simulink model "DTMF_Telefonie_Project_Crehul_Hornai"  (R2018b)
settings: Solver=VariableStepAuto  StartTime=0.0  StopTime=100  RelTol=1e-3
undefined symbols (not defined in the file): fdesignblkfcn, gcbh
libraries: simulink x12, dspfdesign x7
(part 1 of 4)
settings Model: Creator=vladc  LastModifiedBy=vladc

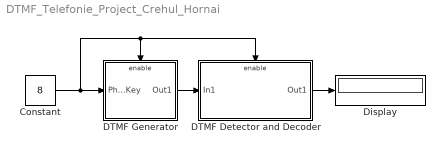
== system DTMF_Telefonie_Project_Crehul_Hornai ==
  Constant : Constant  Value=8  SampleTime=0.00001
  DTMF Detector and Decoder : Subsystem
  DTMF Generator : Subsystem
  Display : Display
      settings: Format=decimal (Stored Integer)
  wires:
  Constant/1 -> DTMF Detector and Decoder/Enable, DTMF Generator/Enable, DTMF Generator/1(PhoneKey)
  DTMF Generator/1(Out1) -> DTMF Detector and Decoder/1(In1)
  DTMF Detector and Decoder/1(Out1) -> Display/1

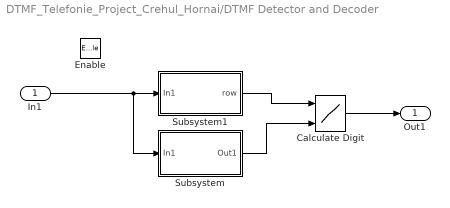
== system DTMF_Telefonie_Project_Crehul_Hornai/DTMF Detector and Decoder ==
  In1 : Inport
  Enable : EnablePort
  Calculate Digit : Lookup_n-D  BreakpointsForDimension1=[1:4]  BreakpointsForDimension2=[1:3]  Table=[1 2 3;4 5 6;7 8 9;10 0 11]  ExtrapMethod=Clip  SaturateOnIntegerOverflow=on  InputSameDT=on
  Subsystem : Subsystem
  Subsystem1 : Subsystem
  Out1 : Outport
  wires:
  In1/1 -> Subsystem/1(In1), Subsystem1/1(In1)
  Calculate Digit/1 -> Out1/1
  Subsystem1/1(row) -> Calculate Digit/1
  Subsystem/1(Out1) -> Calculate Digit/2

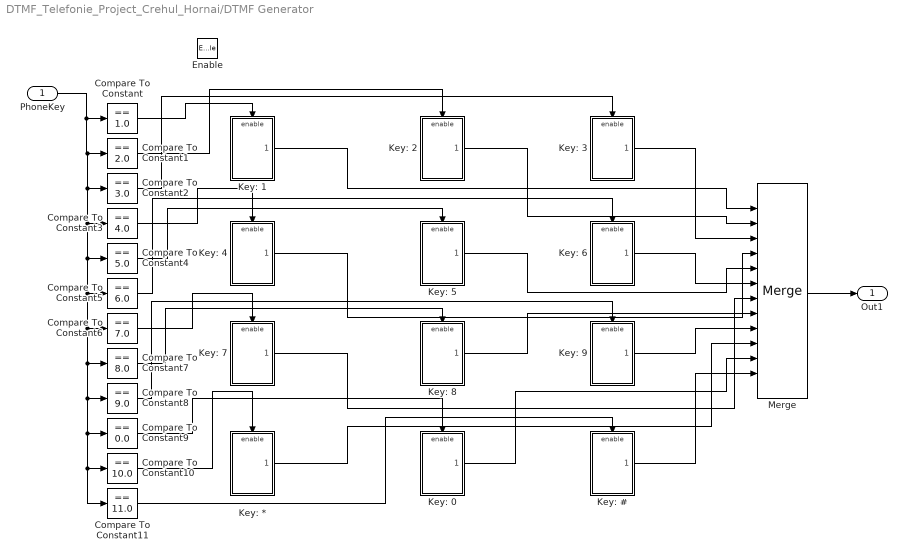
== system DTMF_Telefonie_Project_Crehul_Hornai/DTMF Generator ==
  PhoneKey : Inport
  Enable : EnablePort
  Compare To Constant : simulink/Logic and Bit Operations/Compare To Constant  relop===  const=1.0  OutDataTypeStr=boolean
  Compare To Constant1 : simulink/Logic and Bit Operations/Compare To Constant  relop===  const=2.0  OutDataTypeStr=boolean
  Compare To Constant10 : simulink/Logic and Bit Operations/Compare To Constant  relop===  const=10.0  OutDataTypeStr=boolean
  Compare To Constant11 : simulink/Logic and Bit Operations/Compare To Constant  relop===  const=11.0  OutDataTypeStr=boolean
  Compare To Constant2 : simulink/Logic and Bit Operations/Compare To Constant  relop===  const=3.0  OutDataTypeStr=boolean
  Compare To Constant3 : simulink/Logic and Bit Operations/Compare To Constant  relop===  const=4.0  OutDataTypeStr=boolean
  Compare To Constant4 : simulink/Logic and Bit Operations/Compare To Constant  relop===  const=5.0  OutDataTypeStr=boolean
  Compare To Constant5 : simulink/Logic and Bit Operations/Compare To Constant  relop===  const=6.0  OutDataTypeStr=boolean
  Compare To Constant6 : simulink/Logic and Bit Operations/Compare To Constant  relop===  const=7.0  OutDataTypeStr=boolean
  Compare To Constant7 : simulink/Logic and Bit Operations/Compare To Constant  relop===  const=8.0  OutDataTypeStr=boolean
  Compare To Constant8 : simulink/Logic and Bit Operations/Compare To Constant  relop===  const=9.0  OutDataTypeStr=boolean
  Compare To Constant9 : simulink/Logic and Bit Operations/Compare To Constant  relop===  const=0.0  OutDataTypeStr=boolean
  Key: # : Subsystem
  Key: * : Subsystem
  Key: 0 : Subsystem
  Key: 1 : Subsystem
  Key: 2 : Subsystem
  Key: 3 : Subsystem
  Key: 4 : Subsystem
  Key: 5 : Subsystem
  Key: 6 : Subsystem
  Key: 7 : Subsystem
  Key: 8 : Subsystem
  Key: 9 : Subsystem
  Merge : Merge  Inputs=12
  Out1 : Outport
  wires:
  Key: 7/1(Out_Button_3) -> Merge/7
  PhoneKey/1 -> Compare To Constant11/1, Compare To Constant10/1, Compare To Constant9/1, Compare To Constant8/1, Compare To Constant7/1, Compare To Constant6/1, Compare To Constant5/1, Compare To Constant4/1, Compare To Constant3/1, Compare To Constant2/1, Compare To Constant1/1, Compare To Constant/1
  Compare To Constant6/1 -> Key: 7/Enable
  Key: 1/1(Out_Button_1) -> Merge/1
  Merge/1 -> Out1/1
  Compare To Constant3/1 -> Key: 4/Enable
  Key: 3/1(Out_Button_8) -> Merge/3
  Key: 8/1(Out_Button_7) -> Merge/8
  Compare To Constant4/1 -> Key: 5/Enable
  Key: 0/1(Out_Button_9) -> Merge/11
  Compare To Constant11/1 -> Key: #/Enable
  Compare To Constant/1 -> Key: 1/Enable
  Compare To Constant2/1 -> Key: 3/Enable
  Key: 9/1(Out_Button_11) -> Merge/9
  Compare To Constant9/1 -> Key: 0/Enable
  Compare To Constant10/1 -> Key: */Enable
  Key: 5/1(Out_Button_6) -> Merge/5
  Key: 2/1(Out_Button_5) -> Merge/2
  Key: 6/1(Out_Button_10) -> Merge/6
  Compare To Constant7/1 -> Key: 8/Enable
  Key: */1(Out_Button_4) -> Merge/10
  Compare To Constant5/1 -> Key: 6/Enable
  Compare To Constant8/1 -> Key: 9/Enable
  Compare To Constant1/1 -> Key: 2/Enable
  Key: #/1(Out_Button_12) -> Merge/12
  Key: 4/1(Out_Button_2) -> Merge/4

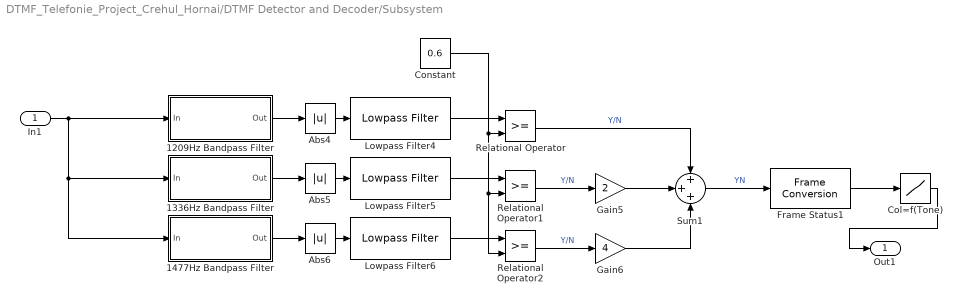
== system DTMF_Telefonie_Project_Crehul_Hornai/DTMF Detector and Decoder/Subsystem ==
  In1 : Inport
  1209Hz Bandpass Filter : Subsystem  DialogController=fdesignblkfcn  InitFcn=fdesignblkfcn(gcbh, {'InitFcn'});  mask(Bandpass Filter){}
      mask help: Design a bandpass filter
      settings: CopyFcn=fdesignblkfcn(gcbh, {'CopyFcn'});
      mask Help: helpview(mapfilelocation('dsp'), 'dspbandpassfilter');
      mask Display: disp('Bandpass');
  1336Hz Bandpass Filter : Subsystem  DialogController=fdesignblkfcn  InitFcn=fdesignblkfcn(gcbh, {'InitFcn'});  mask(Bandpass Filter){}
      mask help: Design a bandpass filter
      settings: CopyFcn=fdesignblkfcn(gcbh, {'CopyFcn'});
      mask Help: helpview(mapfilelocation('dsp'), 'dspbandpassfilter');
      mask Display: disp('Bandpass');
  1477Hz Bandpass Filter : Subsystem  DialogController=fdesignblkfcn  InitFcn=fdesignblkfcn(gcbh, {'InitFcn'});  mask(Bandpass Filter){}
      mask help: Design a bandpass filter
      settings: CopyFcn=fdesignblkfcn(gcbh, {'CopyFcn'});
      mask Help: helpview(mapfilelocation('dsp'), 'dspbandpassfilter');
      mask Display: disp('Bandpass');
  Abs4 : Abs
  Abs5 : Abs
  Abs6 : Abs
  Col=f(Tone) : Lookup_n-D  NumberOfTableDimensions=1  BreakpointsForDimension1=[0:7]  Table=[0 1 2 0 3 0 0 0]  ExtrapMethod=Clip  SaturateOnIntegerOverflow=on  InputSameDT=on
  Constant : Constant  Value=0.6
  Frame Status1 : FrameConversion  OutFrame=Sample-based
  Gain5 : Gain  Gain=2
  Gain6 : Gain  Gain=4
  Lowpass Filter4 : dspfdesign/Lowpass Filter  FilterType=FIR  DesignForMinimumOrder=on  FilterOrder=50  PassbandFrequency=100  StopbandFrequency=130  PassbandRipple=0.1  StopbandAttenuation=80  InheritSampleRate=on  SampleRate=44100  SimulateUsing=Interpreted execution  roundingMode=Floor  coeffsDataTypeStr=fixdt(1,16)
  Lowpass Filter5 : dspfdesign/Lowpass Filter  FilterType=FIR  DesignForMinimumOrder=on  FilterOrder=50  PassbandFrequency=100  StopbandFrequency=130  PassbandRipple=0.1  StopbandAttenuation=80  InheritSampleRate=on  SampleRate=44100  SimulateUsing=Interpreted execution  roundingMode=Floor  coeffsDataTypeStr=fixdt(1,16)
  Lowpass Filter6 : dspfdesign/Lowpass Filter  FilterType=FIR  DesignForMinimumOrder=on  FilterOrder=50  PassbandFrequency=100  StopbandFrequency=130  PassbandRipple=0.1  StopbandAttenuation=80  InheritSampleRate=on  SampleRate=44100  SimulateUsing=Interpreted execution  roundingMode=Floor  coeffsDataTypeStr=fixdt(1,16)
  Relational Operator : RelationalOperator  RndMeth=Nearest  InputSameDT=on
  Relational Operator1 : RelationalOperator  RndMeth=Nearest  InputSameDT=on
  Relational Operator2 : RelationalOperator  RndMeth=Nearest  InputSameDT=on
  Sum1 : Sum  Inputs=+++
  Out1 : Outport
  wires:
  Abs4/1 -> Lowpass Filter4/1
  1336Hz Bandpass Filter/1(Out) -> Abs5/1
  In1/1 -> 1477Hz Bandpass Filter/1(In), 1336Hz Bandpass Filter/1(In), 1209Hz Bandpass Filter/1(In)
  Abs6/1 -> Lowpass Filter6/1
  Abs5/1 -> Lowpass Filter5/1
  1209Hz Bandpass Filter/1(Out) -> Abs4/1
  1477Hz Bandpass Filter/1(Out) -> Abs6/1
  Gain5/1 -> Sum1/2
  Gain6/1 -> Sum1/3
  Sum1/1 -> Frame Status1/1  "YN"
  Frame Status1/1 -> Col=f(Tone)/1
  Col=f(Tone)/1 -> Out1/1
  Lowpass Filter4/1 -> Relational Operator/1
  Lowpass Filter5/1 -> Relational Operator1/1
  Lowpass Filter6/1 -> Relational Operator2/1
  Constant/1 -> Relational Operator2/2, Relational Operator1/2, Relational Operator/2
  Relational Operator/1 -> Sum1/1  "Y/N"
  Relational Operator1/1 -> Gain5/1  "Y/N"
  Relational Operator2/1 -> Gain6/1  "Y/N"

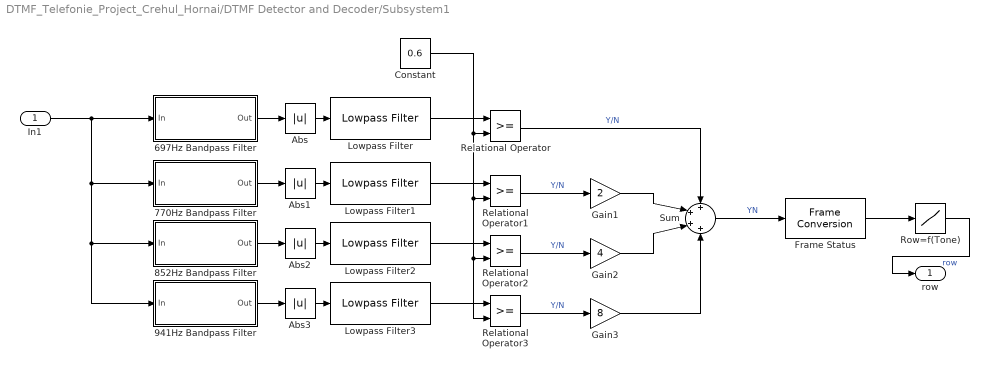
== system DTMF_Telefonie_Project_Crehul_Hornai/DTMF Detector and Decoder/Subsystem1 ==
  In1 : Inport
  697Hz Bandpass Filter : Subsystem  DialogController=fdesignblkfcn  InitFcn=fdesignblkfcn(gcbh, {'InitFcn'});  mask(Bandpass Filter){}
      mask help: Design a bandpass filter
      settings: CopyFcn=fdesignblkfcn(gcbh, {'CopyFcn'});
      mask Help: helpview(mapfilelocation('dsp'), 'dspbandpassfilter');
      mask Display: disp('Bandpass');
  770Hz Bandpass Filter : Subsystem  DialogController=fdesignblkfcn  InitFcn=fdesignblkfcn(gcbh, {'InitFcn'});  mask(Bandpass Filter){}
      mask help: Design a bandpass filter
      settings: CopyFcn=fdesignblkfcn(gcbh, {'CopyFcn'});
      mask Help: helpview(mapfilelocation('dsp'), 'dspbandpassfilter');
      mask Display: disp('Bandpass');
  852Hz Bandpass Filter : Subsystem  DialogController=fdesignblkfcn  InitFcn=fdesignblkfcn(gcbh, {'InitFcn'});  mask(Bandpass Filter){}
      mask help: Design a bandpass filter
      settings: CopyFcn=fdesignblkfcn(gcbh, {'CopyFcn'});
      mask Help: helpview(mapfilelocation('dsp'), 'dspbandpassfilter');
      mask Display: disp('Bandpass');
  941Hz Bandpass Filter : Subsystem  DialogController=fdesignblkfcn  InitFcn=fdesignblkfcn(gcbh, {'InitFcn'});  mask(Bandpass Filter){}
      mask help: Design a bandpass filter
      settings: CopyFcn=fdesignblkfcn(gcbh, {'CopyFcn'});
      mask Help: helpview(mapfilelocation('dsp'), 'dspbandpassfilter');
      mask Display: disp('Bandpass');
  Abs{,1..3} (4 alike) : Abs
  Constant : Constant  Value=0.6
  Frame Status : FrameConversion  OutFrame=Sample-based
  Gain1 : Gain  Gain=2
  Gain2 : Gain  Gain=4
  Gain3 : Gain  Gain=8
  Lowpass Filter : dspfdesign/Lowpass Filter  FilterType=IIR  DesignForMinimumOrder=on  FilterOrder=50  PassbandFrequency=100  StopbandFrequency=230  PassbandRipple=0.1  StopbandAttenuation=20  InheritSampleRate=off  SampleRate=44100  SimulateUsing=Interpreted execution  roundingMode=Floor  coeffsDataTypeStr=fixdt(1,16)
  Lowpass Filter1 : dspfdesign/Lowpass Filter  FilterType=FIR  DesignForMinimumOrder=on  FilterOrder=50  PassbandFrequency=100  StopbandFrequency=130  PassbandRipple=0.1  StopbandAttenuation=80  InheritSampleRate=on  SampleRate=44100  SimulateUsing=Interpreted execution  roundingMode=Floor  coeffsDataTypeStr=fixdt(1,16)
  Lowpass Filter2 : dspfdesign/Lowpass Filter  FilterType=FIR  DesignForMinimumOrder=on  FilterOrder=50  PassbandFrequency=100  StopbandFrequency=130  PassbandRipple=0.1  StopbandAttenuation=80  InheritSampleRate=on  SampleRate=44100  SimulateUsing=Interpreted execution  roundingMode=Floor  coeffsDataTypeStr=fixdt(1,16)
  Lowpass Filter3 : dspfdesign/Lowpass Filter  FilterType=FIR  DesignForMinimumOrder=on  FilterOrder=50  PassbandFrequency=100  StopbandFrequency=130  PassbandRipple=0.1  StopbandAttenuation=80  InheritSampleRate=on  SampleRate=44100  SimulateUsing=Interpreted execution  roundingMode=Floor  coeffsDataTypeStr=fixdt(1,16)
  Relational Operator{,1..3} (4 alike) : RelationalOperator  RndMeth=Nearest  InputSameDT=on
  Row=f(Tone) : Lookup_n-D  NumberOfTableDimensions=1  BreakpointsForDimension1=[0:15]  Table=[0 1 2 0 3 0 0 0 4 0 0 0 0 0 0 0]  ExtrapMethod=Clip  SaturateOnIntegerOverflow=on  InputSameDT=on
  Sum : Sum  Inputs=++++
  row : Outport
  wires:
  Sum/1 -> Frame Status/1  "YN"
  Abs/1 -> Lowpass Filter/1
  Abs1/1 -> Lowpass Filter1/1
  770Hz Bandpass Filter/1(Out) -> Abs1/1
  697Hz Bandpass Filter/1(Out) -> Abs/1
  Abs3/1 -> Lowpass Filter3/1
  Gain2/1 -> Sum/3
  Frame Status/1 -> Row=f(Tone)/1
  Gain3/1 -> Sum/4
  Abs2/1 -> Lowpass Filter2/1
  852Hz Bandpass Filter/1(Out) -> Abs2/1
  941Hz Bandpass Filter/1(Out) -> Abs3/1
  Gain1/1 -> Sum/2
  In1/1 -> 941Hz Bandpass Filter/1(In), 852Hz Bandpass Filter/1(In), 770Hz Bandpass Filter/1(In), 697Hz Bandpass Filter/1(In)
  Row=f(Tone)/1 -> row/1  "row"
  Lowpass Filter/1 -> Relational Operator/1
  Lowpass Filter1/1 -> Relational Operator1/1
  Lowpass Filter2/1 -> Relational Operator2/1
  Lowpass Filter3/1 -> Relational Operator3/1
  Constant/1 -> Relational Operator3/2, Relational Operator2/2, Relational Operator1/2, Relational Operator/2
  Relational Operator/1 -> Sum/1  "Y/N"
  Relational Operator1/1 -> Gain1/1  "Y/N"
  Relational Operator2/1 -> Gain2/1  "Y/N"
  Relational Operator3/1 -> Gain3/1  "Y/N"

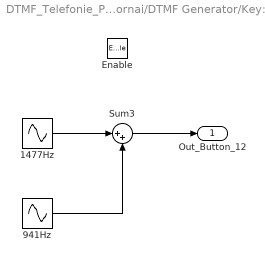
== system DTMF_Telefonie_Project_Crehul_Hornai/DTMF Generator/Key: # ==
  Enable : EnablePort
  1477Hz : Sin  Frequency=1477 * 2 * pi  SampleTime=0.0001
  941Hz : Sin  Frequency=941 * 2 * pi  SampleTime=0.0001
  Sum3 : Sum  Inputs=|++
  Out_Button_12 : Outport
  wires:
  1477Hz/1 -> Sum3/1
  Sum3/1 -> Out_Button_12/1
  941Hz/1 -> Sum3/2

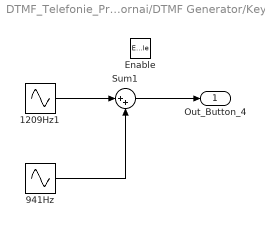
== system DTMF_Telefonie_Project_Crehul_Hornai/DTMF Generator/Key: * ==
  Enable : EnablePort
  1209Hz1 : Sin  Frequency=1209 * 2 * pi  SampleTime=0.0001
  941Hz : Sin  Frequency=941 * 2 * pi  SampleTime=0.0001
  Sum1 : Sum  Inputs=|++
  Out_Button_4 : Outport
  wires:
  941Hz/1 -> Sum1/2
  Sum1/1 -> Out_Button_4/1
  1209Hz1/1 -> Sum1/1

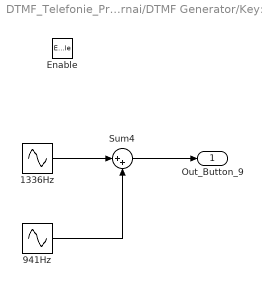
== system DTMF_Telefonie_Project_Crehul_Hornai/DTMF Generator/Key: 0 ==
  Enable : EnablePort
  1336Hz : Sin  Frequency=1336 * 2 * pi  SampleTime=0.0001
  941Hz : Sin  Frequency=941 * 2 * pi  SampleTime=0.0001
  Sum4 : Sum  Inputs=|++
  Out_Button_9 : Outport
  wires:
  1336Hz/1 -> Sum4/1
  Sum4/1 -> Out_Button_9/1
  941Hz/1 -> Sum4/2

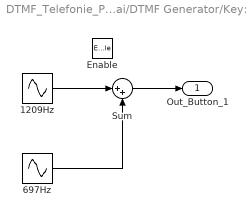
== system DTMF_Telefonie_Project_Crehul_Hornai/DTMF Generator/Key: 1 ==
  Enable : EnablePort
  1209Hz : Sin  Frequency=1209*2*pi  SampleTime=0.0001
  697Hz : Sin  Frequency=697*2*pi  SampleTime=0.0001
  Sum : Sum  Inputs=|++
  Out_Button_1 : Outport
  wires:
  Sum/1 -> Out_Button_1/1
  1209Hz/1 -> Sum/1
  697Hz/1 -> Sum/2

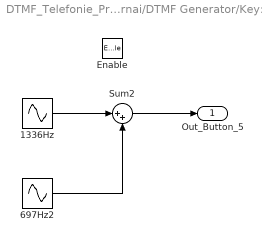
== system DTMF_Telefonie_Project_Crehul_Hornai/DTMF Generator/Key: 2 ==
  Enable : EnablePort
  1336Hz : Sin  Frequency=1336 * 2 * pi  SampleTime=0.0001
  697Hz2 : Sin  Frequency=697 * 2 * pi  SampleTime=0.0001
  Sum2 : Sum  Inputs=|++
  Out_Button_5 : Outport
  wires:
  1336Hz/1 -> Sum2/1
  697Hz2/1 -> Sum2/2
  Sum2/1 -> Out_Button_5/1

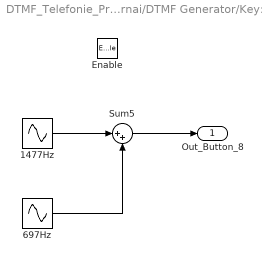
== system DTMF_Telefonie_Project_Crehul_Hornai/DTMF Generator/Key: 3 ==
  Enable : EnablePort
  1477Hz : Sin  Frequency=1477 * 2 * pi  SampleTime=0.0001
  697Hz : Sin  Frequency=697 * 2 * pi  SampleTime=0.0001
  Sum5 : Sum  Inputs=|++
  Out_Button_8 : Outport
  wires:
  697Hz/1 -> Sum5/2
  1477Hz/1 -> Sum5/1
  Sum5/1 -> Out_Button_8/1

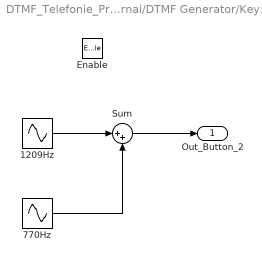
== system DTMF_Telefonie_Project_Crehul_Hornai/DTMF Generator/Key: 4 ==
  Enable : EnablePort
  1209Hz : Sin  Frequency=1209 * 2 * pi  SampleTime=0.0001
  770Hz : Sin  Frequency=770 * 2 * pi  SampleTime=0.0001
  Sum : Sum  Inputs=|++
  Out_Button_2 : Outport
  wires:
  770Hz/1 -> Sum/2
  Sum/1 -> Out_Button_2/1
  1209Hz/1 -> Sum/1

== system DTMF_Telefonie_Project_Crehul_Hornai/DTMF Generator/Key: 5 ==
  Enable : EnablePort
  1336Hz : Sin  Frequency=1336 * 2 * pi  SampleTime=0.0001
  770Hz : Sin  Frequency=770 * 2 * pi  SampleTime=0.0001
  Sum1 : Sum  Inputs=|++
  Out_Button_6 : Outport
  wires:
  Sum1/1 -> Out_Button_6/1
  1336Hz/1 -> Sum1/1
  770Hz/1 -> Sum1/2

== system DTMF_Telefonie_Project_Crehul_Hornai/DTMF Generator/Key: 6 ==
  Enable : EnablePort
  1477Hz : Sin  Frequency=1477 * 2 * pi  SampleTime=0.0001
  770Hz : Sin  Frequency=770 * 2 * pi  SampleTime=0.0001
  Sum1 : Sum  Inputs=|++
  Out_Button_10 : Outport
  wires:
  Sum1/1 -> Out_Button_10/1
  770Hz/1 -> Sum1/2
  1477Hz/1 -> Sum1/1

== system DTMF_Telefonie_Project_Crehul_Hornai/DTMF Generator/Key: 7 ==
  Enable : EnablePort
  1209Hz : Sin  Frequency=1209 * 2 * pi  SampleTime=0.0001
  852Hz : Sin  Frequency=852 * 2 * pi  SampleTime=0.0001
  Sum : Sum  Inputs=|++
  Out_Button_3 : Outport
  wires:
  Sum/1 -> Out_Button_3/1
  852Hz/1 -> Sum/2
  1209Hz/1 -> Sum/1

== system DTMF_Telefonie_Project_Crehul_Hornai/DTMF Generator/Key: 8 ==
  Enable : EnablePort
  1336Hz : Sin  Frequency=1336 * 2 * pi  SampleTime=0.0001
  852Hz : Sin  Frequency=852 * 2 * pi  SampleTime=0.0001
  Sum3 : Sum  Inputs=|++
  Out_Button_7 : Outport
  wires:
  Sum3/1 -> Out_Button_7/1
  852Hz/1 -> Sum3/2
  1336Hz/1 -> Sum3/1

== system DTMF_Telefonie_Project_Crehul_Hornai/DTMF Generator/Key: 9 ==
  Enable : EnablePort
  1477Hz : Sin  Frequency=1477 * 2 * pi  SampleTime=0.0001
  852Hz : Sin  Frequency=852 * 2 * pi  SampleTime=0.0001
  Sum2 : Sum  Inputs=|++
  Out_Button_11 : Outport
  wires:
  1477Hz/1 -> Sum2/1
  Sum2/1 -> Out_Button_11/1
  852Hz/1 -> Sum2/2

== system DTMF_Telefonie_Project_Crehul_Hornai/DTMF Detector and Decoder/Subsystem/1209Hz Bandpass Filter ==
  In : Inport
  Generated Filter Block : DiscreteFir  Tag=BlockMethodSubSystem  Coefficients=[-2.68104316978609227e-05 0.00129524575984109411 0.00027035870583339049 5.97789327057972764e-05 -0.000186064770865025783 -0.00035242675260704643 -0.00033730719511808685 -0.000133492167968419584 0.000159313649341999127 0.00038325330956582161 0.000409612137923090003 0.000213665303268456824 -0.000105208368705157198 -0.000375504388487337922 -0.000447981600112808153 -0.00028128556838711476 3.38150174142128404e-05 0.000324460254122310807 0.000434505373581626424 0.00031190779922032777 3.57001760766895247e-05 -0.000234894518635577658 -0.000355074035898198621 -0.000278061732510660005 -7.37232060620382403e-05 0.00012351148872090335 0.000204887203834534922 0.000153229628683929087 4.43627702712274911e-05 -1.93364116085655968e-05 9.61352545337233223e-06 8.2200891844584666e-05 9.11139960740093863e-05 -3.86869953840555773e-05 -0.000267270539791579281 -0.00043845600455714106 -0.000371517110085582279 -2.57525838629857166e-06 0.000527178747208640773 0.000906762135499263478 0.00082799526502203534 0.000197555808858237633 -0.000736341130457315472 -0.0014631876531442775 -0.00147445872959586473 -0.00060054746165218143 0.000825681716434705166 0.0020556208752338526 0.00231091693758213182 0.00125685357644432115 -0.000720825763344560546 -0.00261642376123233898 -0.00330660983458850406 -0.00219625239510655868 0.000345082450964913118 0.0030589828511720994 0.00440537932230107912 0.00342364119313599662 0.000367194158988320496 -0.00328404793730521912 -0.00552483957470165619 -0.00491298865833330288 -0.00146411400584531997 0.00319144848899657278 0.00655873909436608532 0.00660593914431226777 0.00296540050227270388 -0.00268831680978220749 -0.00738475389415002396 -0.00840901501835418334 -0.00485507173627933251 0.00170278816863107113 0.00787443560336700474 0.0102000406479683427 0.00707754650524016968 -0.000192530533589101833 -0.00790609243381684527 -0.011834345331829723 -0.00953686701253677813 -0.00184357313558901727 0.00737717047285702497 0.0131563591006881898 0.0120995191776441663 0.00436243607936683681 -0.00621715218472063385 -0.0140129083683532656 -0.0146038901566436091 -0.00727232734794326999 0.0043988233791988976 0.0142683352181379036 0.0168697925287066217 0.0104383454868257012 -0.00194538476620552186 -0.013819268353057506 -0.0187150214165393292 -0.013688095887563867 -0.00106668380659103671 0.0126060087320333143 0.0199712647995053949 0.016824321031839895 0.00450931037998957961 -0.0106235729079248737 -0.0204996344955463462 -0.0196414793671116292 -0.00821005216197508332 0.00792476375210000687 0.0202056230547902754 0.0219417901625978823 0.0119644253196142109 -0.00462002904940317372 -0.0190496505763591353 -0.0235536478981206096 -0.0155516191114862881 0.000870680881692380108 0.0170536701314248883 0.0243468151315176726 0.0187524534348275582 0.00312196837493620158 -0.0143009154233129654 -0.0242455404107973886 -0.0213677785659719052 -0.00713308143887335291 0.0109319443381326528 0.0232357829412106198 0.0232357829412106198 0.0109319443381326528 -0.00713308143887335291 -0.0213677785659719052 -0.0242455404107973886 -0.0143009154233129654 0.00312196837493620158 0.0187524534348275582 0.0243468151315176726 0.0170536701314248883 0.000870680881692380108 -0.0155516191114862881 -0.0235536478981206096 -0.0190496505763591353 -0.00462002904940317372 0.0119644253196142109 0.0219417901625978823 0.0202056230547902754 0.00792476375210000687 -0.00821005216197508332 -0.0196414793671116292 -0.0204996344955463462 -0.0106235729079248737 0.00450931037998957961 0.016824321031839895 0.0199712647995053949 0.0126060087320333143 -0.00106668380659103671 -0.013688095887563867 -0.0187150214165393292 -0.013819268353057506 -0.00194538476620552186 0.0104383454868257012 0.0168697925287066217 0.0142683352181379036 0.0043988233791988976 -0.00727232734794326999 -0.0146038901566436091 -0.0140129083683532656 -0.00621715218472063385 0.00436243607936683681 0.0120995191776441663 0.0131563591006881898 0.00737717047285702497 -0.00184357313558901727 -0.00953686701253677813 -0.011834345331829723 ...(+1841 chars)]  InputProcessing=Columns as channels (frame based)
  Out : Outport
  wires:
  In/1 -> Generated Filter Block/1
  Generated Filter Block/1 -> Out/1

== system DTMF_Telefonie_Project_Crehul_Hornai/DTMF Detector and Decoder/Subsystem/1336Hz Bandpass Filter ==
  In : Inport
  Generated Filter Block : DiscreteFir  Tag=BlockMethodSubSystem  Coefficients=[2.69394371099855751e-06 0.00117165562921208344 6.3491850840960342e-05 -8.4624399806407756e-06 -7.99037446358266158e-05 -0.000100868926562373102 -5.44997145059411287e-05 2.99848082026595714e-05 9.79779952662868797e-05 0.000102408748187840688 3.8591008586048468e-05 -5.38855233033176065e-05 -0.000113249385257364584 -9.91491147698982112e-05 -1.76735024774710408e-05 7.81776597637631743e-05 0.000125321473120212782 8.97261386021443435e-05 -6.84389521436474385e-06 -0.000102423933573247061 -0.000132194500866850573 -7.47793614721613091e-05 3.48838671897974944e-05 0.000124265245919175787 0.000133612318573405036 5.35064240703645843e-05 -6.43653826217515952e-05 -0.000142970502120994382 -0.000127873321259458191 -2.73088738157248323e-05 9.45644837702661403e-05 0.000156116735515599145 0.000115425698771689112 -3.70090411639474245e-06 -0.000122933802227524844 -0.000163503928826842218 -9.56295760272910401e-05 3.72712863555299621e-05 0.000149025673371245377 0.000163778588022141236 7.01447106457836044e-05 -7.31253099060873938e-05 -0.000170820259461797229 -0.000157595910391976606 -3.84203641555552668e-05 0.000108265265782551317 0.000186014216685199485 0.000139784366467252596 2.54228694596711317e-06 -0.000141708018935495037 -0.000193703904114099707 -0.000117634172643367625 3.76855386470891472e-05 0.000170912899901319538 0.00019282381288382314 8.69878828140518544e-05 -7.8389945689166839e-05 -0.000194479288599821781 -0.000183199077448570552 -5.02045703261934807e-05 0.000118259217613198844 0.000210623481853642984 0.000164701338875474293 8.73055212596081549e-06 -0.000155018157185409693 -0.000218284554096782359 -0.000137486464077824595 3.52799719571198628e-05 0.000186866881074920213 0.000216201526264954424 0.000102804504377550319 -8.00098318612673959e-05 -0.000211482407583856455 -0.000204360174023499605 -6.17691413268889235e-05 0.000122725198727849242 0.000227685078966525199 0.000182713152657773071 1.67753236851202799e-05 -0.000161565278681012961 -0.000234150769841028191 -0.000152639407700760508 3.0332502399682288e-05 0.000194097650494409919 0.000230632166633668164 0.000114920890391796661 -7.68823833482269823e-05 -0.000218563441804632335 -0.000216183825558373399 -7.13433791556549769e-05 0.000120751682992005938 0.000233377503057401615 0.000192508399706572617 2.48156964049557009e-05 -0.000159397689931879563 -0.000237979533786486291 -0.000159788876706973846 2.29484351225081856e-05 0.000190522502272507917 0.00023167990789653794 0.000120748478138963918 -6.92943979297238038e-05 -0.000212397762841430885 -0.000215371893154697562 -7.66656581665382635e-05 0.000110994915730187101 0.000224468546324539881 0.000189426814851585213 3.08040640945889555e-05 -0.000146479066566603932 -0.000225473033556930578 -0.000156045409631158909 1.47784474854167902e-05 0.000173213119583249088 0.000216116279365059435 0.000116843378449837162 -5.67977950993890299e-05 -0.000190310363448117914 -0.000196786541266158205 -7.49770548206403747e-05 9.32354527198771005e-05 0.000196623409868828918 0.000169673649135869365 3.2817692787847361e-05 -0.000121481738994366675 -0.000192623660969485364 -0.000136337989629350953 6.44294111745713494e-06 0.000140439368990387522 0.000178501959768861355 9.97765686525447452e-05 -4.05829609781086648e-05 -0.000148761926126928477 -0.000156468179317936253 -6.27785878042827743e-05 6.66565411803262536e-05 0.000146855225949184048 0.000128144911822030381 2.8422048619754876e-05 -8.36632672263093197e-05 -0.000134813266803125503 -9.67845224833618466e-05 4.76836132450508474e-07 8.99481120179559598e-05 0.000114987091168748971 6.50792747704405632e-05 -2.12987572827511538e-05 -8.56772032055124616e-05 -8.92309014011464716e-05 -3.66047012556492291e-05 3.22993008562691072e-05 7.15226375672178491e-05 6.06921033006627229e-05 1.42402568271595819e-05 -3.21240483136897657e-05 -4.93228887105787335e-05 -3.25150958583107601e-05 -9.98438621711752322e-07 2.08458830929236782e-05 2.13769857401605382e-05 8.64939430702377741e-06 -1.20579606564959717e-06 1.03140375700815773e-06 ...(+19722 chars)]  InputProcessing=Columns as channels (frame based)
  Out : Outport
  wires:
  In/1 -> Generated Filter Block/1
  Generated Filter Block/1 -> Out/1
